simulink model "antiwindup"  (R2023b)
settings: Solver=VariableStepAuto  StartTime=0.0  StopTime=5  RelTol=1e-3
values from neighbouring files (symbols this model uses):
  AccionDirecta = 0    [windup.m]
  consigna = 100    [windup.m]
  InicioEstimador = 10    [windup.m]
  kamp = 1    [windup.m]
undefined symbols (not defined in the file or in its folder): C, ke0, Kid, Ld, p0, sysd, T
libraries: simulink x2
settings Model: Creator=erwinplanck  LastModifiedBy=erwinplanck

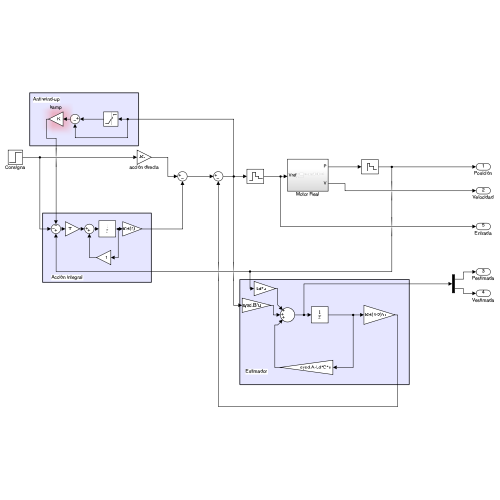
[thumbnail: Simulink's stored preview of the top-level diagram]
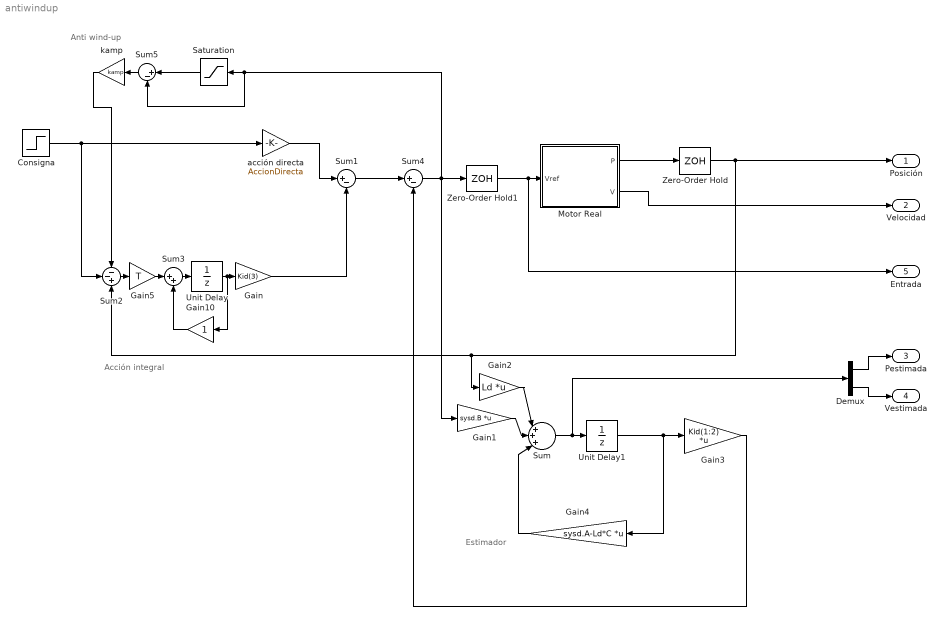
== system antiwindup ==
  note: Anti wind-up
  note: Estimador
  note: Acción integral
  Consigna : Step  Time=0.01  After=consigna  SampleTime=0
  Demux : Demux  Outputs=2
  Gain : Gain  Gain=Kid(3)
  Gain1 : Gain  Gain=sysd.B  Multiplication=Matrix(K*u)
  Gain10 : Gain
  Gain2 : Gain  Gain=Ld  Multiplication=Matrix(K*u)
  Gain3 : Gain  Gain=Kid(1:2)  Multiplication=Matrix(K*u)
  Gain4 : Gain  Gain=sysd.A-Ld*C  Multiplication=Matrix(K*u)
  Gain5 : Gain  Gain=T
  Motor Real : Subsystem
  Saturation : Saturate  UpperLimit=12  LowerLimit=-12
  Sum : Sum  Inputs=|+++|
  Sum1 : Sum  Inputs=|+-
  Sum2 : Sum  Inputs=--+
  Sum3 : Sum  Inputs=|++
  Sum4 : Sum  Inputs=|+-
  Sum5 : Sum  Inputs=|+-
  Unit Delay : UnitDelay  SampleTime=T  HasFrameUpgradeWarning=on
  Unit Delay1 : UnitDelay  InitialCondition=InicioEstimador  SampleTime=T  HasFrameUpgradeWarning=on
  Zero-Order Hold : ZeroOrderHold  SampleTime=T
  Zero-Order Hold1 : ZeroOrderHold  SampleTime=T
  acción directa : Gain  Gain=AccionDirecta
  kamp : Gain  Gain=kamp
  Posición : Outport
  Velocidad : Outport  Port=2
  Pestimada : Outport  Port=3
  Vestimada : Outport  Port=4
  Entrada : Outport  Port=5
  wires:
  Sum3/1 -> Unit Delay/1
  Gain4/1 -> Sum/3
  Sum1/1 -> Sum4/1
  Gain3/1 -> Sum4/2
  Consigna/1 -> acción directa/1, Sum2/2
  Gain/1 -> Sum1/2
  acción directa/1 -> Sum1/1
  Motor Real/1(P) -> Zero-Order Hold/1
  Gain1/1 -> Sum/2
  Gain10/1 -> Sum3/2
  Unit Delay1/1 -> Gain4/1, Gain3/1
  Sum2/1 -> Gain5/1
  Gain5/1 -> Sum3/1
  Gain2/1 -> Sum/1
  Unit Delay/1 -> Gain10/1, Gain/1
  Sum4/1 -> Gain1/1, Sum5/2, Saturation/1, Zero-Order Hold1/1
  Saturation/1 -> Sum5/1
  Sum5/1 -> kamp/1
  kamp/1 -> Sum2/1
  Zero-Order Hold/1 -> Posición/1, Sum2/3, Gain2/1
  Motor Real/2(V) -> Velocidad/1
  Sum/1 -> Demux/1, Unit Delay1/1
  Demux/2 -> Vestimada/1
  Demux/1 -> Pestimada/1
  Zero-Order Hold1/1 -> Entrada/1, Motor Real/1(Vref)

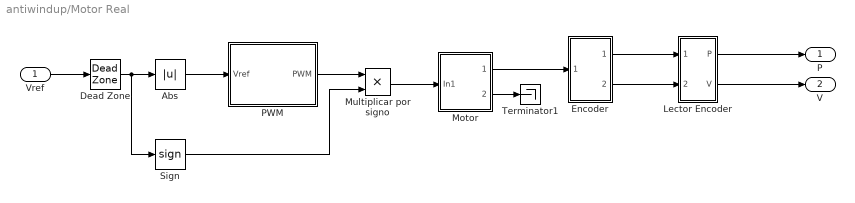
== system antiwindup/Motor Real ==
  Vref : Inport
  " Multiplicar por signo" : Product
  Abs : Abs  SaturateOnIntegerOverflow=off
  Dead Zone : DeadZone  LowerValue=-0.2  UpperValue=0.2
  Encoder : Subsystem
  Lector Encoder : Subsystem
  Motor : Subsystem
  PWM : Subsystem  mask{T=0.001, Vmax=12}
      mask prompts: T "Periodo"; Vmax "Voltaje"
  Sign : Signum
  Terminator1 : Terminator
  P : Outport
  V : Outport  Port=2
  wires:
  Encoder/1("Enc1 ") -> Lector Encoder/1(Enc1)
  Lector Encoder/1(P) -> P/1
  Motor/2(Velocidad) -> Terminator1/1
  Lector Encoder/2(V) -> V/1
  Vref/1 -> Dead Zone/1
  Dead Zone/1 -> Sign/1, Abs/1
  Encoder/2("Enc2 ") -> Lector Encoder/2(Enc2)
  Sign/1 -> " Multiplicar por signo"/2
  Motor/1(Posición) -> Encoder/1(Pos)
  " Multiplicar por signo"/1 -> Motor/1(In1)
  Abs/1 -> PWM/1(Vref)
  PWM/1(PWM) -> " Multiplicar por signo"/1

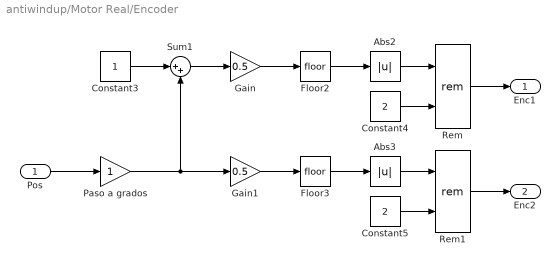
== system antiwindup/Motor Real/Encoder ==
  Pos : Inport
  Abs2 : Abs  SaturateOnIntegerOverflow=off
  Abs3 : Abs  SaturateOnIntegerOverflow=off
  Constant3 : Constant
  Constant4 : Constant  Value=2
  Constant5 : Constant  Value=2
  Floor2 : Rounding
  Floor3 : Rounding
  Gain : Gain  Gain=0.5
  Gain1 : Gain  Gain=0.5
  Paso a grados : Gain
  Rem : Math  Operator=rem
  Rem1 : Math  Operator=rem
  Sum1 : Sum  Inputs=|++
  "Enc1 " : Outport  SampleTime=0.0001
  "Enc2 " : Outport  Port=2  SampleTime=0.0001
  wires:
  Gain/1 -> Floor2/1
  Rem1/1 -> "Enc2 "/1
  Abs2/1 -> Rem/1
  Pos/1 -> Paso a grados/1
  Abs3/1 -> Rem1/1
  Paso a grados/1 -> Gain1/1, Sum1/2
  Constant5/1 -> Rem1/2
  Constant3/1 -> Sum1/1
  Constant4/1 -> Rem/2
  Floor2/1 -> Abs2/1
  Rem/1 -> "Enc1 "/1
  Floor3/1 -> Abs3/1
  Sum1/1 -> Gain/1
  Gain1/1 -> Floor3/1

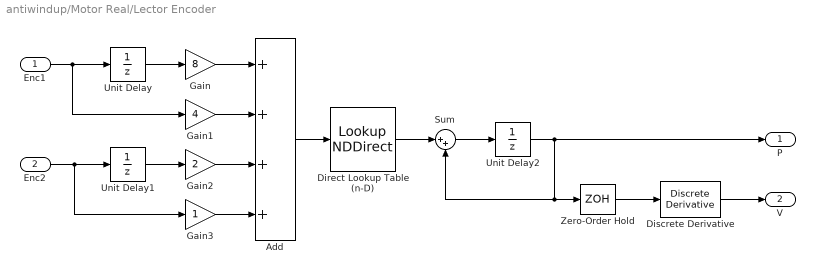
== system antiwindup/Motor Real/Lector Encoder ==
  Enc1 : Inport
  Enc2 : Inport  Port=2
  Add : Sum  Inputs=++++  OutDataTypeStr=double
  Direct Lookup Table (n-D) : LookupNDDirect  NumberOfTableDimensions=1  Table=[0,-1,1,0,1,0,0,-1,-1,0,0,1,0,1,-1,0]
  Discrete Derivative : simulink/Discrete/Discrete Derivative  gainval=1.0  ICPrevScaledInput=0.0  OutMin=[]  OutMax=[]  OutDataType=fixdt(1, 16)  OutScaling=2^-10  DoSatur=off
  Gain : Gain  Gain=8
  Gain1 : Gain  Gain=4
  Gain2 : Gain  Gain=2
  Gain3 : Gain
  Sum : Sum  Inputs=|++
  Unit Delay : UnitDelay  SampleTime=-1  HasFrameUpgradeWarning=on
  Unit Delay1 : UnitDelay  SampleTime=-1  HasFrameUpgradeWarning=on
  Unit Delay2 : UnitDelay  SampleTime=-1  HasFrameUpgradeWarning=on
  Zero-Order Hold : ZeroOrderHold  SampleTime=0.01
  P : Outport
  V : Outport  Port=2
  wires:
  Unit Delay/1 -> Gain/1
  Add/1 -> Direct Lookup Table (n-D)/1
  Enc2/1 -> Unit Delay1/1, Gain3/1
  Gain/1 -> Add/1
  Unit Delay2/1 -> Zero-Order Hold/1, Sum/2, P/1
  Gain1/1 -> Add/2
  Enc1/1 -> Unit Delay/1, Gain1/1
  Unit Delay1/1 -> Gain2/1
  Gain2/1 -> Add/3
  Discrete Derivative/1 -> V/1
  Gain3/1 -> Add/4
  Direct Lookup Table (n-D)/1 -> Sum/1
  Sum/1 -> Unit Delay2/1
  Zero-Order Hold/1 -> Discrete Derivative/1

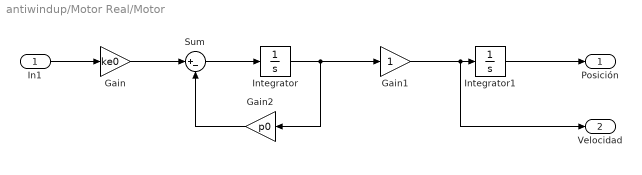
== system antiwindup/Motor Real/Motor ==
  In1 : Inport
  Gain : Gain  Gain=ke0
  Gain1 : Gain
  Gain2 : Gain  Gain=p0
  Integrator : Integrator
  Integrator1 : Integrator
  Sum : Sum  Inputs=|+-
  Posición : Outport
  Velocidad : Outport  Port=2
  wires:
  Gain/1 -> Sum/1
  Sum/1 -> Integrator/1
  Integrator/1 -> Gain2/1, Gain1/1
  In1/1 -> Gain/1
  Gain1/1 -> Velocidad/1, Integrator1/1
  Gain2/1 -> Sum/2
  Integrator1/1 -> Posición/1

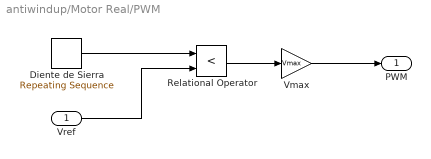
== system antiwindup/Motor Real/PWM ==
  Vref : Inport
  "Diente de Sierra " : simulink/Sources/Repeating Sequence  rep_seq_t=linspace(0, T, 100)  rep_seq_y=linspace(0,Vmax,100)
  Relational Operator : RelationalOperator  Operator=<  OutDataTypeStr=boolean  RndMeth=Simplest  InputSameDT=off
  Vmax : Gain  Gain=Vmax
  PWM : Outport
  wires:
  Vmax/1 -> PWM/1
  Vref/1 -> Relational Operator/2
  "Diente de Sierra "/1 -> Relational Operator/1
  Relational Operator/1 -> Vmax/1
